simulink model "comparetoconstant_test_tmp"  (Simulink 8.3)
settings: Solver=ode45  StartTime=0.0  StopTime=10.0  RelTol=1e-3
libraries: simulink x13
settings Model: Creator=arnaud  LastModifiedBy=hbourbou
settings DataIOCC: SaveFormat=Structure  SignalLoggingSaveFormat=Dataset
settings DebuggingCC: UnderspecifiedInitializationDetection=Simplified  MergeDetectMultiDrivingBlocksExec=error  FrameProcessingCompatibilityMsg=error  StateNameClashWarn=none
settings GRTTargetCC: CombineOutputUpdateFcns=on  GRTInterface=off

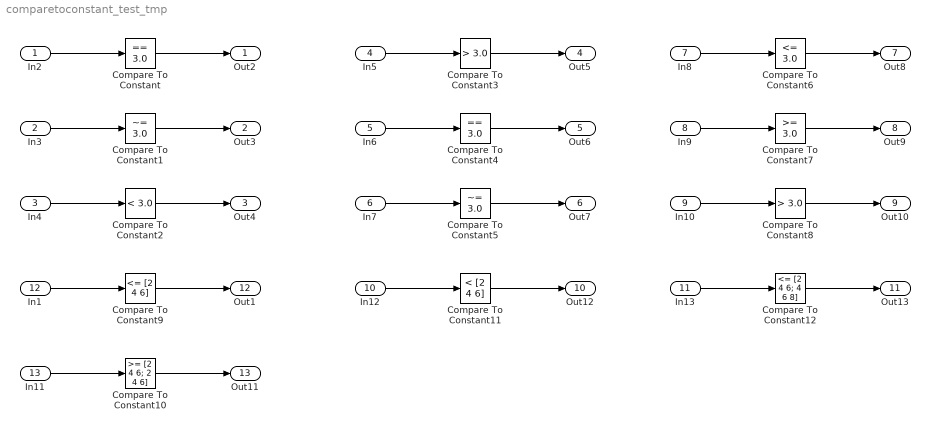
== system comparetoconstant_test_tmp ==
  In2 : Inport  OutDataTypeStr=double
  In3 : Inport  Port=2  OutDataTypeStr=int8
  In4 : Inport  Port=3  OutDataTypeStr=boolean
  In5 : Inport  Port=4  OutDataTypeStr=double  PortDimensions=3
  In6 : Inport  Port=5  OutDataTypeStr=int8  PortDimensions=3
  In7 : Inport  Port=6  OutDataTypeStr=boolean  PortDimensions=3
  In8 : Inport  Port=7  OutDataTypeStr=double  PortDimensions=[2 3]
  In9 : Inport  Port=8  OutDataTypeStr=int8  PortDimensions=[2 3]
  In10 : Inport  Port=9  OutDataTypeStr=boolean  PortDimensions=[2 3]
  In12 : Inport  Port=10  OutDataTypeStr=double  PortDimensions=3
  In13 : Inport  Port=11  OutDataTypeStr=double  PortDimensions=[2 3]
  In1 : Inport  Port=12  OutDataTypeStr=double
  In11 : Inport  Port=13  OutDataTypeStr=double
  Compare To Constant : simulink/Logic and Bit Operations/Compare To Constant  relop===  const=3.0  OutDataTypeStr=boolean
  Compare To Constant1 : simulink/Logic and Bit Operations/Compare To Constant  relop=~=  const=3.0  OutDataTypeStr=boolean
  Compare To Constant10 : simulink/Logic and Bit Operations/Compare To Constant  relop=>=  const=[2 4 6; 2 4 6]  OutDataTypeStr=boolean
  Compare To Constant11 : simulink/Logic and Bit Operations/Compare To Constant  relop=<  const=[2 4 6]  OutDataTypeStr=boolean
  Compare To Constant12 : simulink/Logic and Bit Operations/Compare To Constant  relop=<=  const=[2 4 6; 4 6 8]  OutDataTypeStr=boolean
  Compare To Constant2 : simulink/Logic and Bit Operations/Compare To Constant  relop=<  const=3.0  OutDataTypeStr=boolean
  Compare To Constant3 : simulink/Logic and Bit Operations/Compare To Constant  relop=>  const=3.0  OutDataTypeStr=boolean
  Compare To Constant4 : simulink/Logic and Bit Operations/Compare To Constant  relop===  const=3.0  OutDataTypeStr=boolean
  Compare To Constant5 : simulink/Logic and Bit Operations/Compare To Constant  relop=~=  const=3.0  OutDataTypeStr=boolean
  Compare To Constant6 : simulink/Logic and Bit Operations/Compare To Constant  relop=<=  const=3.0  OutDataTypeStr=boolean
  Compare To Constant7 : simulink/Logic and Bit Operations/Compare To Constant  relop=>=  const=3.0  OutDataTypeStr=boolean
  Compare To Constant8 : simulink/Logic and Bit Operations/Compare To Constant  relop=>  const=3.0  OutDataTypeStr=boolean
  Compare To Constant9 : simulink/Logic and Bit Operations/Compare To Constant  relop=<=  const=[2 4 6]  OutDataTypeStr=boolean
  Out2 : Outport
  Out3 : Outport  Port=2
  Out4 : Outport  Port=3
  Out5 : Outport  Port=4
  Out6 : Outport  Port=5
  Out7 : Outport  Port=6
  Out8 : Outport  Port=7
  Out9 : Outport  Port=8
  Out10 : Outport  Port=9
  Out12 : Outport  Port=10
  Out13 : Outport  Port=11
  Out1 : Outport  Port=12
  Out11 : Outport  Port=13
  wires:
  Compare To Constant/1 -> Out2/1
  In2/1 -> Compare To Constant/1
  Compare To Constant1/1 -> Out3/1
  In3/1 -> Compare To Constant1/1
  Compare To Constant2/1 -> Out4/1
  In4/1 -> Compare To Constant2/1
  Compare To Constant3/1 -> Out5/1
  In5/1 -> Compare To Constant3/1
  Compare To Constant4/1 -> Out6/1
  In6/1 -> Compare To Constant4/1
  Compare To Constant5/1 -> Out7/1
  In7/1 -> Compare To Constant5/1
  Compare To Constant6/1 -> Out8/1
  In8/1 -> Compare To Constant6/1
  Compare To Constant7/1 -> Out9/1
  In9/1 -> Compare To Constant7/1
  Compare To Constant8/1 -> Out10/1
  In10/1 -> Compare To Constant8/1
  Compare To Constant11/1 -> Out12/1
  In12/1 -> Compare To Constant11/1
  Compare To Constant12/1 -> Out13/1
  In13/1 -> Compare To Constant12/1
  Compare To Constant9/1 -> Out1/1
  In1/1 -> Compare To Constant9/1
  Compare To Constant10/1 -> Out11/1
  In11/1 -> Compare To Constant10/1
